simulink model "proyecto"  (R2018a)
settings: Solver=VariableStepAuto  StartTime=0.0  StopTime=10.0  RelTol=1e-3
values from neighbouring files (symbols this model uses):
  alpha = (1-sin(phin))/(sin(phin)+1)    [practica5.m]    (also in proyectoAvilaSilva.m = (1-(sin(teta)))/(1+(sin(teta))); proyectoAvilaSilva2.m = (1-(sin(teta)))/(1+(sin(teta))))
  K = 1.1    [Practica2Oscar.m]    (also in proyectoAvilaSilva.m = Kp/limite; proyectoAvilaSilva2.m = Kp/limite)
  T = 2.5    [P4OscarAvilaControlDigital.m]    (also in Practica2Oscar.m = 1; practica5.m = 0.02; proyectoAvilaSilva.m = 0.01; proyectoAvilaSilva2.m = 0.01)
  tao = 1/(vm*sqrt(alpha))    [practica5.m]    (also in proyectoAvilaSilva.m; proyectoAvilaSilva2.m)
settings Model: Creator=sasm  LastModifiedBy=Oscar

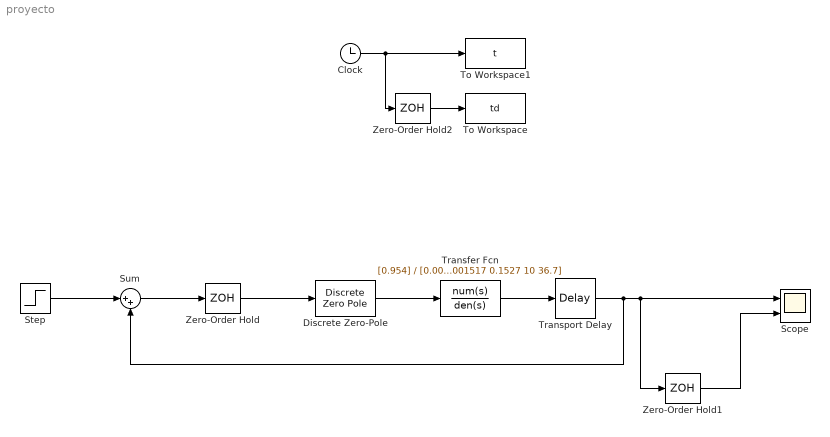
== system proyecto ==
  Clock : Clock
  Discrete Zero-Pole : DiscreteZeroPole  Zeros=[-1/tao]  Poles=[-1/(tao*alpha)]  Gain=K  SampleTime=T
  Scope : Scope  NumInputPorts=2
  Step : Step  SampleTime=T
  Sum : Sum  Inputs=|++
  To Workspace : ToWorkspace  VariableName=td  SaveFormat=Timeseries  SampleTime=T
  To Workspace1 : ToWorkspace  VariableName=t  SampleTime=T
  Transfer Fcn : TransferFcn  Numerator=[0.954]  Denominator=[0.00001517 0.1527 10 36.7]
  Transport Delay : TransportDelay  DelayTime=0.1
  Zero-Order Hold : ZeroOrderHold  SampleTime=T
  Zero-Order Hold1 : ZeroOrderHold  SampleTime=T
  Zero-Order Hold2 : ZeroOrderHold  SampleTime=T
  wires:
  Step/1 -> Sum/1
  Sum/1 -> Zero-Order Hold/1
  Zero-Order Hold/1 -> Discrete Zero-Pole/1
  Discrete Zero-Pole/1 -> Transfer Fcn/1
  Transfer Fcn/1 -> Transport Delay/1
  Zero-Order Hold1/1 -> Scope/2
  Transport Delay/1 -> Sum/2, Zero-Order Hold1/1, Scope/1
  Clock/1 -> Zero-Order Hold2/1, To Workspace1/1
  Zero-Order Hold2/1 -> To Workspace/1
